simulink model "mconversionFixPointSupport3"  (Simulink 8.0)
settings: Solver=ode5  StartTime=0.0  StopTime=30  RelTol=1e-3
settings Model: Creator=The Mathworks Inc.  LastModifiedBy=htu  ExtModeAutoUpdateStatusClock=off
settings DataIOCC: SignalLoggingSaveFormat=ModelDataLogs  SignalLoggingName=logsOut
settings OptimizationCC: InlineParams=on  InlineInvariantSignals=on  InitFltsAndDblsToZero=on
settings DebuggingCC: SaveWithParameterizedLinksMsg=none  CheckExecutionContextPreStartOutputMsg=on  CheckExecutionContextRuntimeOutputMsg=on  SignalResolutionControl=TryResolveAllWithWarning  SolverPrmCheckMsg=none  MultiTaskDSMMsg=warning  MultiTaskCondExecSysMsg=none
settings HardwareCC: ProdHWDeviceType=Specified  TargetHWDeviceType=32-bit Generic  ProdEqTarget=off
settings ModelReferenceCC: UpdateModelReferenceTargets=IfOutOfDate
settings RTWCC: ProcessScript=grt_make_rtw_hook  IncludeERTFirstTime=on
settings GRTTargetCC: TargetFcnLib=ansi_tfl_tmw.mat  CombineOutputUpdateFcns=off  GRTInterface=on

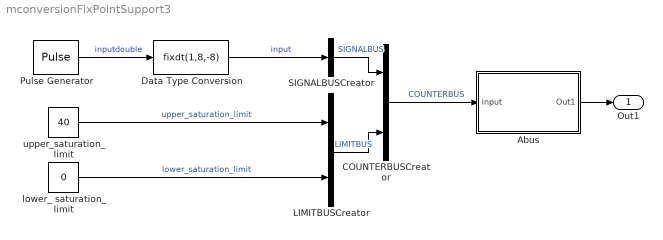
== system mconversionFixPointSupport3 ==
  Abus : Subsystem  TreatAsAtomicUnit=on
  COUNTERBUSCreator : BusCreator  DialogController=Simulink.DDGSource_Bus  Inputs=2
  Data Type Conversion : DataTypeConversion  OutDataTypeStr=fixdt(1,8,-8)
  LIMITBUSCreator : BusCreator  DialogController=Simulink.DDGSource_Bus  Inputs=2
  Pulse Generator : DiscretePulseGenerator  Amplitude=int32(1)  SampleTime=0.1
  SIGNALBUSCreator : BusCreator  DialogController=Simulink.DDGSource_Bus  Inputs=1
  lower_ saturation_ limit : Constant  Value=0  OutDataTypeStr=fixdt(1,8,-8)  SampleTime=0.1
  upper_saturation_limit : Constant  Value=40  OutDataTypeStr=fixdt(1,8,-8)  SampleTime=0.1
  Out1 : Outport
  wires:
  upper_saturation_limit/1 -> LIMITBUSCreator/1  "upper_saturation_limit"
  LIMITBUSCreator/1 -> COUNTERBUSCreator/2  "LIMITBUS"
  Pulse Generator/1 -> Data Type Conversion/1  "inputdouble"
  COUNTERBUSCreator/1 -> Abus/1(" input")  "COUNTERBUS"
  Abus/1(Out1) -> Out1/1
  SIGNALBUSCreator/1 -> COUNTERBUSCreator/1  "SIGNALBUS"
  Data Type Conversion/1 -> SIGNALBUSCreator/1  "input"
  lower_ saturation_ limit/1 -> LIMITBUSCreator/2  "lower_saturation_limit"

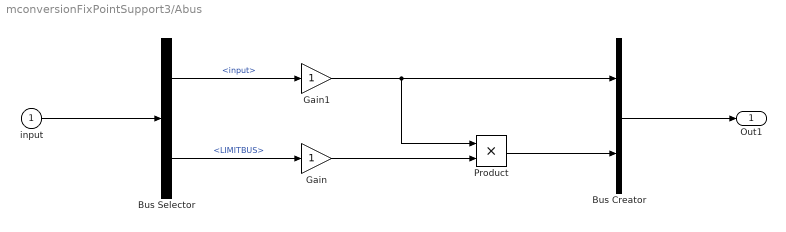
== system mconversionFixPointSupport3/Abus ==
  " input" : Inport
  Bus Creator : BusCreator  DialogController=Simulink.DDGSource_Bus  Inputs=2
  Bus Selector : BusSelector  DialogController=Simulink.DDGSource_Bus  OutputSignals=SIGNALBUS.input,LIMITBUS
  Gain : Gain  ParamDataTypeStr=Inherit: Same as input
  Gain1 : Gain  ParamDataTypeStr=Inherit: Same as input
  Product : Product  RndMeth=Zero  OutDataTypeStr=Inherit: Same as first input
  Out1 : Outport
  wires:
  Bus Selector/2 -> Gain/1  "<LIMITBUS>"
  Bus Creator/1 -> Out1/1
  Bus Selector/1 -> Gain1/1  "<input>"
  Gain1/1 -> Bus Creator/1, Product/1
  " input"/1 -> Bus Selector/1
  Gain/1 -> Product/2
  Product/1 -> Bus Creator/2
